simulink model "uz_mpc_cost_and_optim_state_machine"  (R2021a)
settings: Solver=FixedStepAuto  StartTime=0.0  StopTime=10000*t_ADC  RelTol=1e-3
values from neighbouring files (symbols this model uses):
  A = 1.0    (= 1)    [uz_6ph_pu_vsd_voltages_init.m]    (also in uz_mpc_6ph_init.m; uz_mpc_6ph_state_machine_init.m = 0.1)
  f = n_rpm/60.0*p    (= 250)    [uz_6ph_pu_vsd_voltages_init.m]    (also in uz_mpc_6ph_init.m; uz_mpc_6ph_state_machine_init.m = 83.3333333333)
  IB = sqrt(2)*IR    [uz_6ph_pu_vsd_voltages_init.m]    (also in uz_mpc_6ph_init.m; uz_mpc_6ph_state_machine_init.m)
  id_ref = 0.0    (= 0)    [uz_6ph_pu_vsd_voltages_init.m]    (also in uz_mpc_6ph_init.m; uz_mpc_6ph_state_machine_init.m)
  iq_ref = -10.0    (= -10)    [uz_6ph_pu_vsd_voltages_init.m]    (also in uz_mpc_6ph_init.m; uz_mpc_6ph_state_machine_init.m = 5)
  ix_ref = 0.0    (= 0)    [uz_6ph_pu_vsd_voltages_init.m]    (also in uz_mpc_6ph_init.m; uz_mpc_6ph_state_machine_init.m)
  iy_ref = 0.0    (= 0)    [uz_6ph_pu_vsd_voltages_init.m]    (also in uz_mpc_6ph_init.m; uz_mpc_6ph_state_machine_init.m)
  lambda_d = 1.0    (= 1)    [uz_mpc_6ph_state_machine_init.m]
  lambda_q = 1.0    (= 1)    [uz_mpc_6ph_state_machine_init.m]
  lambda_u = 0.0    (= 0)    [uz_mpc_6ph_state_machine_init.m]
  lambda_x = 0.1    [uz_mpc_6ph_state_machine_init.m]
  lambda_y = 0.1    [uz_mpc_6ph_state_machine_init.m]
  Ld_over_LB = Ld/LB    [uz_6ph_pu_vsd_voltages_init.m]    (also in uz_mpc_6ph_init.m; uz_mpc_6ph_state_machine_init.m)
  Lq_over_LB = Lq/LB    [uz_6ph_pu_vsd_voltages_init.m]    (also in uz_mpc_6ph_init.m; uz_mpc_6ph_state_machine_init.m)
  n_rpm = 3000    [uz_6ph_pu_vsd_voltages_init.m]    (also in uz_mpc_6ph_init.m; uz_mpc_6ph_state_machine_init.m = 1000)
  omega_m = n_rpm*pi/30    (= 314.159265359)    [uz_6ph_pu_vsd_voltages_init.m]    (also in uz_mpc_6ph_init.m; uz_mpc_6ph_state_machine_init.m = 104.71975512)
  omegaB = nR*2*pi()/60*p    [uz_6ph_pu_vsd_voltages_init.m]    (also in uz_mpc_6ph_init.m; uz_mpc_6ph_state_machine_init.m)
  p = 5    [uz_6ph_pu_vsd_voltages_init.m]    (also in uz_mpc_6ph_init.m; uz_mpc_6ph_state_machine_init.m)
  psi_pm_over_psiB = psi_pm/psiB    [uz_6ph_pu_vsd_voltages_init.m]    (also in uz_mpc_6ph_init.m; uz_mpc_6ph_state_machine_init.m)
  Rs_over_ZB = Rs/ZB    [uz_6ph_pu_vsd_voltages_init.m]    (also in uz_mpc_6ph_init.m; uz_mpc_6ph_state_machine_init.m)
  t_ADC = 1/f_ADC    (= 1e-05)    [uz_6ph_pu_vsd_voltages_init.m]    (also in uz_mpc_6ph_init.m; uz_mpc_6ph_state_machine_init.m; uz_typeconv_init.m)
  t_clock = 1/f_clock    (= 1e-08)    [uz_6ph_pu_vsd_voltages_init.m]    (also in uz_mpc_6ph_init.m; uz_mpc_6ph_state_machine_init.m; uz_typeconv_init.m)
  Ts_times_ZB_over_Ld = Ts*ZB/Ld    [uz_6ph_pu_vsd_voltages_init.m]    (also in uz_mpc_6ph_init.m; uz_mpc_6ph_state_machine_init.m)
  Ts_times_ZB_over_Lq = Ts*ZB/Lq    [uz_6ph_pu_vsd_voltages_init.m]    (also in uz_mpc_6ph_init.m; uz_mpc_6ph_state_machine_init.m)
  Ts_times_ZB_over_Lx = Ts*ZB/Lx    [uz_6ph_pu_vsd_voltages_init.m]    (also in uz_mpc_6ph_init.m; uz_mpc_6ph_state_machine_init.m)
  Ts_times_ZB_over_Ly = Ts*ZB/Ly    [uz_6ph_pu_vsd_voltages_init.m]    (also in uz_mpc_6ph_init.m; uz_mpc_6ph_state_machine_init.m)
  v_dc = 565.0    (= 565)    [uz_6ph_pu_vsd_voltages_init.m]    (also in uz_mpc_6ph_init.m; uz_mpc_6ph_state_machine_init.m)
  VB = sqrt(2/3)*VR    [uz_6ph_pu_vsd_voltages_init.m]    (also in uz_mpc_6ph_init.m; uz_mpc_6ph_state_machine_init.m)
libraries: nesl_utility x38, fl_lib x30, ee_lib x14, simulink x10, hdlsllib x2
(part 3 of 3)

== matlab function uz_mpc_cost_and_optim_state_machine/uz_6ph_mpc_pu_voltages_vsd/finite_control_set ==
  settings: fimath=fimath('RoundingMethod', 'Floor','OverflowAction', 'Wrap','ProductMode', 'FullPrecision', 'SumMode', 'FullPrecision')
  data: v_DC_pu input; sin_angle input; pu_ud output; pu_uq output; pu_ux output; pu_uy output; cos_angle input; index input
function [pu_ud,pu_uq,pu_ux,pu_uy] = voltage_space_vectors(v_DC_pu, sin_angle, cos_angle, index)

fm = fimath();
v_DC_pu = fi(v_DC_pu,1,18,15,fm);
sin_angle = fi(sin_angle,1,18,16,fm);
cos_angle = fi(cos_angle,1,18,16,fm);

% u_d-voltages lookup factors alpha/beta
vd_pu = fi([0.000000,  0.000000;
0.333333,  -0.000000;
-0.166667,  0.288675;
0.166667,  0.288675;
-0.166667,  -0.288675;
0.166667,  -0.288675;
-0.333333,  0.000000;
0.000000,  0.000000;
0.288675,  0.166667;
0.622008,  0.166667;
0.122008,  0.455342;
0.455342,  0.455342;
0.122008,  -0.122008;
0.455342,  -0.122008;
-0.044658,  0.166667;
0.288675,  0.166667;
-0.288675,  0.166667;
0.044658,  0.166667;
-0.455342,  0.455342;
-0.122008,  0.455342;
-0.455342,  -0.122008;
-0.122008,  -0.122008;
-0.622008,  0.166667;
-0.288675,  0.166667;
0.000000,  0.333333;
0.333333,  0.333333;
-0.166667,  0.622008;
0.166667,  0.622008;
-0.166667,  0.044658;
0.166667,  0.044658;
-0.333333,  0.333333;
0.000000,  0.333333;
-0.000000,  -0.333333;
0.333333,  -0.333333;
-0.166667,  -0.044658;
0.166667,  -0.044658;
-0.166667,  -0.622008;
0.166667,  -0.622008;
-0.333333,  -0.333333;
-0.000000,  -0.333333;
0.288675,  -0.166667;
0.622008,  -0.166667;
0.122008,  0.122008;
0.455342,  0.122008;
0.122008,  -0.455342;
0.455342,  -0.455342;
-0.044658,  -0.166667;
0.288675,  -0.166667;
-0.288675,  -0.166667;
0.044658,  -0.166667;
-0.455342,  0.122008;
-0.122008,  0.122008;
-0.455342,  -0.455342;
-0.122008,  -0.455342;
-0.622008,  -0.166667;
-0.288675,  -0.166667;
0.000000,  0.000000;
0.333333,  -0.000000;
-0.166667,  0.288675;
0.166667,  0.288675;
-0.166667,  -0.288675;
0.166667,  -0.288675;
-0.333333,  0.000000;
0.000000,  0.000000],1,18,15);

% u_q-voltages lookup factors alpha/beta
vq_pu = fi([0.000000, 0.000000;
0.333333, -0.000000;
-0.166667, 0.288675;
0.166667, 0.288675;
-0.166667, -0.288675;
0.166667, -0.288675;
-0.333333, 0.000000;
0.000000, 0.000000;
0.288675, 0.166667;
0.622008, 0.166667;
0.122008, 0.455342;
0.455342, 0.455342;
0.122008, -0.122008;
0.455342, -0.122008;
-0.044658, 0.166667;
0.288675, 0.166667;
-0.288675, 0.166667;
0.044658, 0.166667;
-0.455342, 0.455342;
-0.122008, 0.455342;
-0.455342, -0.122008;
-0.122008, -0.122008;
-0.622008, 0.166667;
-0.288675, 0.166667;
0.000000, 0.333333;
0.333333, 0.333333;
-0.166667, 0.622008;
0.166667, 0.622008;
-0.166667, 0.044658;
0.166667, 0.044658;
-0.333333, 0.333333;
0.000000, 0.333333;
-0.000000, -0.333333;
0.333333, -0.333333;
-0.166667, -0.044658;
0.166667, -0.044658;
-0.166667, -0.622008;
0.166667, -0.622008;
-0.333333, -0.333333;
-0.000000, -0.333333;
0.288675, -0.166667;
0.622008, -0.166667;
0.122008, 0.122008;
0.455342, 0.122008;
0.122008, -0.455342;
0.455342, -0.455342;
-0.044658, -0.166667;
0.288675, -0.166667;
-0.288675, -0.166667;
0.044658, -0.166667;
-0.455342, 0.122008;
-0.122008, 0.122008;
-0.455342, -0.455342;
-0.122008, -0.455342;
-0.622008, -0.166667;
-0.288675, -0.166667;
0.000000, 0.000000;
0.333333, -0.000000;
-0.166667, 0.288675;
0.166667, 0.288675;
-0.166667, -0.288675;
0.166667, -0.288675;
-0.333333, 0.000000;
0.000000, 0.000000],1,18,15);
     
% u_x-voltages
vx_pu = fi([0.000000;
0.333333;
-0.166667;
0.166667;
-0.166667;
0.166667;
-0.333333;
0.000000;
-0.288675;
0.044658;
-0.455342;
-0.122008;
-0.455342;
-0.122008;
-0.622008;
-0.288675;
0.288675;
0.622008;
0.122008;
0.455342;
0.122008;
0.455342;
-0.044658;
0.288675;
0.000000;
0.333333;
-0.166667;
0.166667;
-0.166667;
0.166667;
-0.333333;
0.000000;
-0.000000;
0.333333;
-0.166667;
0.166667;
-0.166667;
0.166667;
-0.333333;
-0.000000;
-0.288675;
0.044658;
-0.455342;
-0.122008;
-0.455342;
-0.122008;
-0.622008;
-0.288675;
0.288675;
0.622008;
0.122008;
0.455342;
0.122008;
0.455342;
-0.044658;
0.288675;
0.000000;
0.333333;
-0.166667;
0.166667;
-0.166667;
0.166667;
-0.333333;
0.000000],1,18,15);

% u_y-voltages
vy_pu = fi([0.000000;
-0.000000;
-0.288675;
-0.288675;
0.288675;
0.288675;
0.000000;
0.000000;
0.166667;
0.166667;
-0.122008;
-0.122008;
0.455342;
0.455342;
0.166667;
0.166667;
0.166667;
0.166667;
-0.122008;
-0.122008;
0.455342;
0.455342;
0.166667;
0.166667;
0.333333;
0.333333;
0.044658;
0.044658;
0.622008;
0.622008;
0.333333;
0.333333;
-0.333333;
-0.333333;
-0.622008;
-0.622008;
-0.044658;
-0.044658;
-0.333333;
-0.333333;
-0.166667;
-0.166667;
-0.455342;
-0.455342;
0.122008;
0.122008;
-0.166667;
-0.166667;
-0.166667;
-0.166667;
-0.455342;
-0.455342;
0.122008;
0.122008;
-0.166667;
-0.166667;
0.000000;
-0.000000;
-0.288675;
-0.288675;
0.288675;
0.288675;
0.000000;
0.000000],1,18,15);

pu_ud = fi(v_DC_pu * (vd_pu(index,1) * cos_angle + vd_pu(index,2) * sin_angle),1,27,24);
pu_uq = fi(v_DC_pu * (vq_pu(index,1) * -sin_angle + vq_pu(index,2) * cos_angle),1,27,24);
pu_ux = fi(v_DC_pu * vx_pu(index),1,27,24);
pu_uy = fi(v_DC_pu * vy_pu(index),1,27,24);

== matlab function uz_mpc_cost_and_optim_state_machine/uz_vsd_6ph_30deg/VSD_6ph_30deg ==
  settings: fimath=fimath('RoundingMethod', 'Floor','OverflowAction', 'Wrap','ProductMode', 'FullPrecision', 'SumMode', 'FullPrecision')
  data: a1 input; alpha output; b1 input; c1 input; a2 input; b2 input; c2 input; beta output; x1 output; y1 output; z1 output; z2 output
function [alpha,beta,x1,y1,z1,z2] = fcn(a1,b1,c1,a2,b2,c2)


A = [fi(0,1,18,11) fi(0,1,18,11) fi(0,1,18,11) fi(0,1,18,11) fi(0,1,18,11) fi(0,1,18,11)]';

A =    2/6*[1    -0.5        -0.5        sqrt(3)/2   -sqrt(3)/2  0 ;
           0    sqrt(3)/2   -sqrt(3)/2  0.5         0.5         -1;
           1    -0.5        -0.5        -sqrt(3)/2  sqrt(3)/2   0 ;
           0    -sqrt(3)/2  sqrt(3)/2   0.5         0.5         -1;
           0.5   0.5          0.5          0           0           0 ;
           0    0           0           0.5          0.5          0.5] * [a1 b1 c1 a2 b2 c2]';

alpha = fi(A(1),1,18,11);
beta = fi(A(2),1,18,11);
x1 = fi(A(3),1,18,11);
y1 = fi(A(4),1,18,11);
z1 = fi(A(5),1,18,11);
z2 = fi(A(6),1,18,11);

== matlab function uz_mpc_cost_and_optim_state_machine/uz_6ph_mpc_costs_and_optimization/MATLAB Function ==
  settings: fimath=fimath('RoundingMethod', 'Floor','OverflowAction', 'Wrap','ProductMode', 'FullPrecision', 'SumMode', 'FullPrecision')
  data: in input; G_next output; index input; last_optim_index input; G_prev output
function [G_next,G_prev] = get_switch_positions(in,index,last_optim_index)
%#codegen
G_next = in(index,[1 3 5 7 9 11]);
G_prev = in(last_optim_index,[1 3 5 7 9 11]);

== matlab function uz_mpc_cost_and_optim_state_machine/uz_6ph_mpc_costs_and_optimization/iterativesearch ==
  data: index input; opt_idx output; cost input; min_costs output
function [opt_idx,min_costs] = fcn(index, cost)
%#codegen

persistent cost_old
if isempty(cost_old)
    cost_old = fi(4.98,0,27,24);
end

persistent index_old
if isempty(index_old)
    index_old = uint8(1);
end

persistent opt_idx_old
if isempty(opt_idx_old)
    opt_idx_old = uint8(1);
end


if (index < 63)       
       
if (index ~= index_old)
   if (cost <= cost_old)
       opt_idx_old = index; 
       cost_old = cost;
   else
    
    
   end
   index_old = index;
end

else
       cost_old = fi(4.98,0,27,24);
end

min_costs = cost_old;
opt_idx = opt_idx_old;

== matlab function uz_mpc_cost_and_optim_state_machine/uz_6ph_mpc_costs_and_optimization/FiniteControlSetSwitchingTable ==
  settings: fimath=fimath('RoundingMethod', 'Floor','OverflowAction', 'Wrap','ProductMode', 'FullPrecision', 'SumMode', 'FullPrecision')
  data: G output
function G  = switchingTable

% -------------------------------------------------------------------
%  Generated by MATLAB on 14-Oct-2020 14:52:37
%  MATLAB version: 9.4.0.813654 (R2018a)
% -------------------------------------------------------------------
                                         

s1_v = boolean([0; 1; 0; 1; 0; 1; 0; 1; 0; 1; 0; 1; 0; 1; 0; 1; 0; 1; 0; 1; 0; ...
        1; 0; 1; 0; 1; 0; 1; 0; 1; 0; 1; 0; 1; 0; 1; 0; 1; 0; 1; 0; 1; ...
        0; 1; 0; 1; 0; 1; 0; 1; 0; 1; 0; 1; 0; 1; 0; 1; 0; 1; 0; 1; 0; ...
        1]);


s2_v = boolean([1; 0; 1; 0; 1; 0; 1; 0; 1; 0; 1; 0; 1; 0; 1; 0; 1; 0; 1; 0; 1; ...
        0; 1; 0; 1; 0; 1; 0; 1; 0; 1; 0; 1; 0; 1; 0; 1; 0; 1; 0; 1; 0; ...
        1; 0; 1; 0; 1; 0; 1; 0; 1; 0; 1; 0; 1; 0; 1; 0; 1; 0; 1; 0; 1; ...
        0]);


s3_v = boolean([0; 0; 1; 1; 0; 0; 1; 1; 0; 0; 1; 1; 0; 0; 1; 1; 0; 0; 1; 1; 0; ...
        0; 1; 1; 0; 0; 1; 1; 0; 0; 1; 1; 0; 0; 1; 1; 0; 0; 1; 1; 0; 0; ...
        1; 1; 0; 0; 1; 1; 0; 0; 1; 1; 0; 0; 1; 1; 0; 0; 1; 1; 0; 0; 1; ...
        1]);


s4_v = boolean([1; 1; 0; 0; 1; 1; 0; 0; 1; 1; 0; 0; 1; 1; 0; 0; 1; 1; 0; 0; 1; ...
        1; 0; 0; 1; 1; 0; 0; 1; 1; 0; 0; 1; 1; 0; 0; 1; 1; 0; 0; 1; 1; ...
        0; 0; 1; 1; 0; 0; 1; 1; 0; 0; 1; 1; 0; 0; 1; 1; 0; 0; 1; 1; 0; ...
        0]);


s5_v = boolean([0; 0; 0; 0; 1; 1; 1; 1; 0; 0; 0; 0; 1; 1; 1; 1; 0; 0; 0; 0; 1; ...
        1; 1; 1; 0; 0; 0; 0; 1; 1; 1; 1; 0; 0; 0; 0; 1; 1; 1; 1; 0; 0; ...
        0; 0; 1; 1; 1; 1; 0; 0; 0; 0; 1; 1; 1; 1; 0; 0; 0; 0; 1; 1; 1; ...
        1]);


s6_v = boolean([1; 1; 1; 1; 0; 0; 0; 0; 1; 1; 1; 1; 0; 0; 0; 0; 1; 1; 1; 1; 0; ...
        0; 0; 0; 1; 1; 1; 1; 0; 0; 0; 0; 1; 1; 1; 1; 0; 0; 0; 0; 1; 1; ...
        1; 1; 0; 0; 0; 0; 1; 1; 1; 1; 0; 0; 0; 0; 1; 1; 1; 1; 0; 0; 0; ...
        0]);


s7_v = boolean([0; 0; 0; 0; 0; 0; 0; 0; 1; 1; 1; 1; 1; 1; 1; 1; 0; 0; 0; 0; 0; ...
        0; 0; 0; 1; 1; 1; 1; 1; 1; 1; 1; 0; 0; 0; 0; 0; 0; 0; 0; 1; 1; ...
        1; 1; 1; 1; 1; 1; 0; 0; 0; 0; 0; 0; 0; 0; 1; 1; 1; 1; 1; 1; 1; ...
        1]);


s8_v = boolean([1; 1; 1; 1; 1; 1; 1; 1; 0; 0; 0; 0; 0; 0; 0; 0; 1; 1; 1; 1; 1; ...
        1; 1; 1; 0; 0; 0; 0; 0; 0; 0; 0; 1; 1; 1; 1; 1; 1; 1; 1; 0; 0; ...
        0; 0; 0; 0; 0; 0; 1; 1; 1; 1; 1; 1; 1; 1; 0; 0; 0; 0; 0; 0; 0; ...
        0]);


s9_v = boolean([0; 0; 0; 0; 0; 0; 0; 0; 0; 0; 0; 0; 0; 0; 0; 0; 1; 1; 1; 1; 1; ...
        1; 1; 1; 1; 1; 1; 1; 1; 1; 1; 1; 0; 0; 0; 0; 0; 0; 0; 0; 0; 0; ...
        0; 0; 0; 0; 0; 0; 1; 1; 1; 1; 1; 1; 1; 1; 1; 1; 1; 1; 1; 1; 1; ...
        1]);


s10_v = boolean([1; 1; 1; 1; 1; 1; 1; 1; 1; 1; 1; 1; 1; 1; 1; 1; 0; 0; 0; 0; 0; ...
         0; 0; 0; 0; 0; 0; 0; 0; 0; 0; 0; 1; 1; 1; 1; 1; 1; 1; 1; 1; 1; ...
         1; 1; 1; 1; 1; 1; 0; 0; 0; 0; 0; 0; 0; 0; 0; 0; 0; 0; 0; 0; 0; ...
         0]);


s11_v = boolean([0; 0; 0; 0; 0; 0; 0; 0; 0; 0; 0; 0; 0; 0; 0; 0; 0; 0; 0; 0; 0; ...
         0; 0; 0; 0; 0; 0; 0; 0; 0; 0; 0; 1; 1; 1; 1; 1; 1; 1; 1; 1; 1; ...
         1; 1; 1; 1; 1; 1; 1; 1; 1; 1; 1; 1; 1; 1; 1; 1; 1; 1; 1; 1; 1; ...
         1]);


s12_v = boolean([1; 1; 1; 1; 1; 1; 1; 1; 1; 1; 1; 1; 1; 1; 1; 1; 1; 1; 1; 1; 1; ...
         1; 1; 1; 1; 1; 1; 1; 1; 1; 1; 1; 0; 0; 0; 0; 0; 0; 0; 0; 0; 0; ...
         0; 0; 0; 0; 0; 0; 0; 0; 0; 0; 0; 0; 0; 0; 0; 0; 0; 0; 0; 0; 0; ...
         0]);
     
G = [s1_v, s2_v, s3_v, s4_v, s5_v, s6_v, s7_v, s8_v, s9_v, s10_v, s11_v, s12_v];
